simulink model "NoiseComparison"  (Simulink 6.3)
settings: Solver=FixedStepDiscrete  StartTime=0.0  StopTime=1000  FixedStep=Tp  MaxStep=0.01  RelTol=1e-3
values from neighbouring files (symbols this model uses):
  Tp = 0.001    [CW1_3a_skrypt.m]    (also in CW1_3c_skrypt.m; CW1_3d_skrypt.m; CW2_1a_skrypt.m; CW2_1b_skrypt.m)
libraries: simulink x1
settings Model: LastModifiedBy=szymon

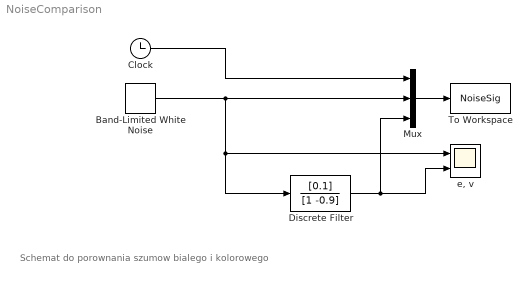
== system NoiseComparison ==
  note: Schemat do porownania szumow bialego i kolorowego
  Band-Limited White Noise : simulink/Sources/Band-Limited White Noise  Cov=[10]  Ts=Tp  seed=[23341]
  Clock : Clock
      settings: Decimation=10
  Discrete Filter : DiscreteFilter  Numerator=[0.1]  Denominator=[1 -0.9]  SampleTime=Tp
  Mux : Mux  Inputs=3
  To Workspace : ToWorkspace  VariableName=NoiseSig  SampleTime=-1  SaveFormat=Array
  "e, v" : Scope  NumInputPorts=2
      settings: TimeRange=1000  YMin=-15~-3  YMax=15~3
  wires:
  Mux/1 -> To Workspace/1
  Clock/1 -> Mux/1
  Band-Limited White Noise/1 -> Mux/2, Discrete Filter/1, "e, v"/1
  Discrete Filter/1 -> Mux/3, "e, v"/2
